simulink model "testNmpcPred_sim"  (R2022a)
settings: Solver=FixedStepAuto  StartTime=0.0  StopTime=0.5  FixedStep=0.01  RelTol=1e-3
values from neighbouring files (symbols this model uses):
  N = 12    [pred_val_data.mat]    (also in testNmpcPred.m)
  q0 = [-1.19464003762e-05 6.7750855603e-06 -9.11003216872e-06 -1.8284628242e-05 -2.65504111959e-05 -1.27617776572e-05 -0.000131356264542 1.04702440163 -1.74424979698 -0.882000293112 -0.00236266084125 -2.1946749064]    [pred_val_data.mat]    (also in testNmpcPred.m = xTT(seconds(0), :).xk(1:N))
  q_dot_0 = [-4.7789426306e-05 2.70806007007e-05 -3.64231556994e-05 -7.25882000905e-05 -0.000106683779215 -5.10494341622e-05 -0.0005213817664 -0.000695584891458 0.00431643119192 -0.0372746195538 -0.00967509504595 -8.77865586758]    [pred_val_data.mat]    (also in testNmpcPred.m = xTT(seconds(0), :).xk(N+7:2*N+6))
  xee0 = [3.55203644097 -0.2 1.3362227665 0 0 0]    [pred_val_data.mat]    (also in testNmpcPred.m = xTT(seconds(0), :).xk(N+1:N+6))
  xee_dot_0 = xTT(seconds(0), :).xk(2*N+7:2*N+12)    [testNmpcPred.m]
settings Model: Creator=charl  LastModifiedBy=charl

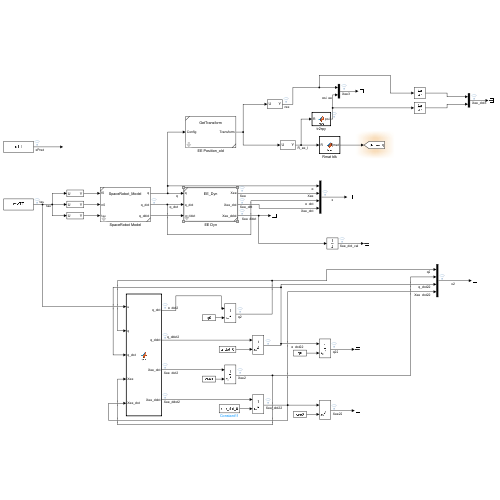
[thumbnail: Simulink's stored preview of the top-level diagram]
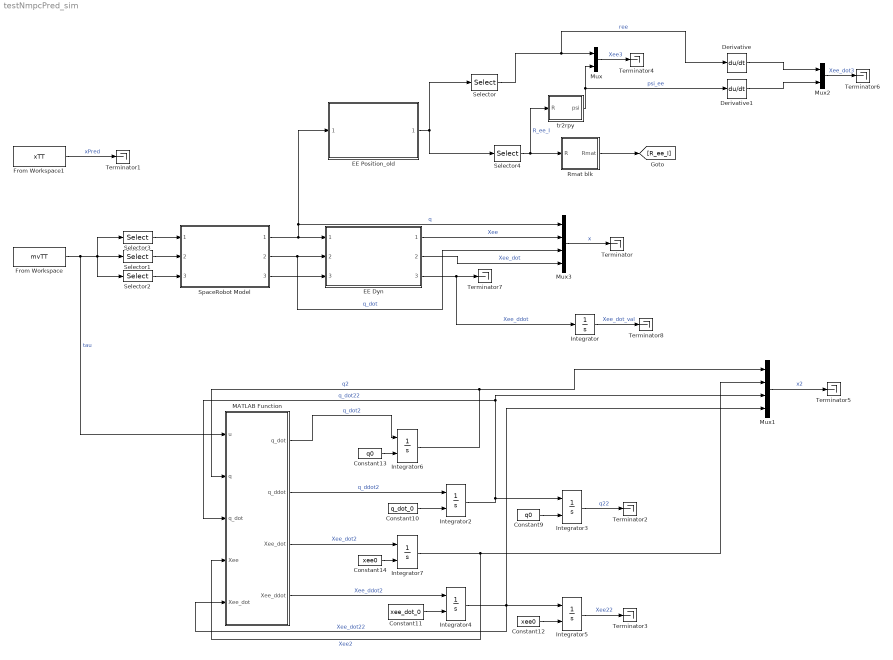
== system testNmpcPred_sim ==
  Constant10 : Constant  Value=q_dot_0
  Constant11 : Constant  Value=xee_dot_0
  Constant12 : Constant  Value=xee0
  Constant13 : Constant  Value=q0
  Constant14 : Constant  Value=xee0
  Constant9 : Constant  Value=q0
  Derivative : Derivative
  Derivative1 : Derivative
  EE Dyn : Subsystem  ReferencedSubsystem=EE_Dyn  spaceRobot=sr
  EE Position_old : Subsystem  ReferencedSubsystem=GetTransform  spaceRobot=sr  sourceBody=endeffector  targetBody=inertial  SimulateUsing=Interpreted execution
  From Workspace : FromWorkspace  VariableName=mvTT
  From Workspace1 : FromWorkspace  VariableName=xTT
  Integrator : Integrator  InitialCondition=xee_dot_0'
  Integrator{2..7} (6 alike) : Integrator  InitialConditionSource=external
  MATLAB Function : MATLAB Function  TreatAsAtomicUnit=on
  Mux : Mux  Inputs=2
  Mux1 : Mux
  Mux2 : Mux  Inputs=2
  Mux3 : Mux
  Rmat blk : MATLAB Function  TreatAsAtomicUnit=on
  Selector : Selector  NumberOfDimensions=2  InputPortWidth=[4 4]  IndexOptions=Index vector (dialog),Index vector (dialog)  Indices=[1:3],4  OutputSizes=1,1
  Selector1 : Selector  IndexOptions=Index vector (dialog)  Indices=[4:6]  OutputSizes=1
  Selector2 : Selector  IndexOptions=Index vector (dialog)  Indices=[7:N]  OutputSizes=1
  Selector3 : Selector  IndexOptions=Index vector (dialog)  Indices=[1:3]  OutputSizes=1
  Selector4 : Selector  NumberOfDimensions=2  InputPortWidth=[4 4]  IndexOptions=Index vector (dialog),Index vector (dialog)  Indices=[1:3],[1:3]  OutputSizes=1,1
  SpaceRobot Model : Subsystem  ReferencedSubsystem=SpaceRobot_Model  spaceRobot=sr  jointCstr=off  q_0=q0  q_dot_0=q_dot_0
  Terminator{,1..8} (9 alike) : Terminator
  tr2rpy : MATLAB Function  TreatAsAtomicUnit=on
  wires:
  Selector3/1 -> SpaceRobot Model/1
  From Workspace/1 -> MATLAB Function/1(u), Selector2/1, Selector1/1, Selector3/1  "tau"
  Selector2/1 -> SpaceRobot Model/3
  Selector1/1 -> SpaceRobot Model/2
  EE Dyn/2 -> Mux3/4  "Xee_dot"
  SpaceRobot Model/2 -> Mux3/3, EE Dyn/2  "q_dot"
  SpaceRobot Model/1 -> EE Dyn/1, EE Position_old/1, Mux3/1  "q"
  Mux3/1 -> Terminator/1  "x"
  EE Dyn/1 -> Mux3/2  "Xee"
  From Workspace1/1 -> Terminator1/1  "xPred"
  Constant9/1 -> Integrator3/2
  Integrator6/1 -> Mux1/1, MATLAB Function/2(q)  "q2"
  MATLAB Function/4(Xee_ddot) -> Integrator4/1  "Xee_ddot2"
  Constant12/1 -> Integrator5/2
  Integrator3/1 -> Terminator2/1  "q22"
  Integrator7/1 -> MATLAB Function/4(Xee), Mux1/2  "Xee2"
  Constant10/1 -> Integrator2/2
  Integrator2/1 -> Integrator3/1, Mux1/3, MATLAB Function/3("q_dot ")  "q_dot22"
  Constant13/1 -> Integrator6/2
  MATLAB Function/2(q_ddot) -> Integrator2/1  "q_ddot2"
  MATLAB Function/3(Xee_dot) -> Integrator7/1  "Xee_dot2"
  MATLAB Function/1(q_dot) -> Integrator6/1  "q_dot2"
  Integrator5/1 -> Terminator3/1  "Xee22"
  Constant14/1 -> Integrator7/2
  Integrator4/1 -> Mux1/4, Integrator5/1, MATLAB Function/5("Xee_dot ")  "Xee_dot22"
  Constant11/1 -> Integrator4/2
  Mux1/1 -> Terminator5/1  "x2"
  EE Position_old/1 -> Selector4/1, Selector/1
  Selector/1 -> Derivative/1, Mux/1  "ree"
  Rmat blk/1(Rmat) -> [R_ee_I]
  Selector4/1 -> tr2rpy/1(R), Rmat blk/1(R)  "R_ee_I"
  tr2rpy/1(psi) -> Derivative1/1, Mux/2  "psi_ee"
  Mux/1 -> Terminator4/1  "Xee3"
  Mux2/1 -> Terminator6/1  "Xee_dot3"
  Derivative/1 -> Mux2/1
  Derivative1/1 -> Mux2/2
  SpaceRobot Model/3 -> EE Dyn/3
  EE Dyn/3 -> Integrator/1, Terminator7/1  "Xee_ddot"
  Integrator/1 -> Terminator8/1  "Xee_dot_val"

== matlab function testNmpcPred_sim/MATLAB Function ==
  data: u input; q_dot output; q input; q_ddot output; Xee_dot output; q_dot input; Xee input; Xee_dot input; Xee_ddot output
function [q_dot, q_ddot, Xee_dot, Xee_ddot] = fcn(u, q, q_dot, Xee, Xee_dot)

q_dot(4:6) = omega2euler(q(4:6), q_dot(4:6));
Xee_dot(4:6) = omega2euler(Xee(4:6), Xee_dot(4:6));

x = [q; Xee; q_dot; Xee_dot];

% sr_info = SR2_info();
sr_info = SR6_info();


N = sr_info.N;

dx = sr_ee_state_func(x, u, sr_info);

% q_dot = dx(1:8);
% q_ddot = dx(15:22);
% 
% Xee_dot = dx(9:14);
% Xee_ddot = dx(23:28);

q_dot = dx(1:N);
q_ddot = dx(N+7:2*N+6);

Xee_dot = dx(N+1:N+6);
Xee_ddot = dx(end-5:end);

== matlab function testNmpcPred_sim/Rmat blk ==
  data: R input; Rmat output
function Rmat = fcn(R)

Rmat = blkdiag(R, R);

== matlab function testNmpcPred_sim/tr2rpy ==
  data: R input; psi output size=[3, 1]
function psi = fcn(R)
% Computes euler angle from rotation matrix

psi = zeros(3, 1);

temp = rotm2eul(R, 'ZYX');
psi(1) = temp(3);
psi(2) = temp(2);
psi(3) = temp(1);
